simulink library "INT_TIntkVUs_DD"  (R2016b)
settings: Solver=VariableStepAuto  StartTime=0.0  StopTime=10.0  RelTol=1e-3
settings Model: Creator=Administrator  LastModifiedBy=Administrator

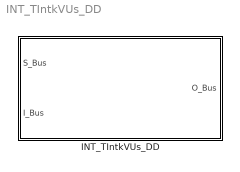
== system INT_TIntkVUs_DD ==
  INT_TIntkVUs_DD : Subsystem

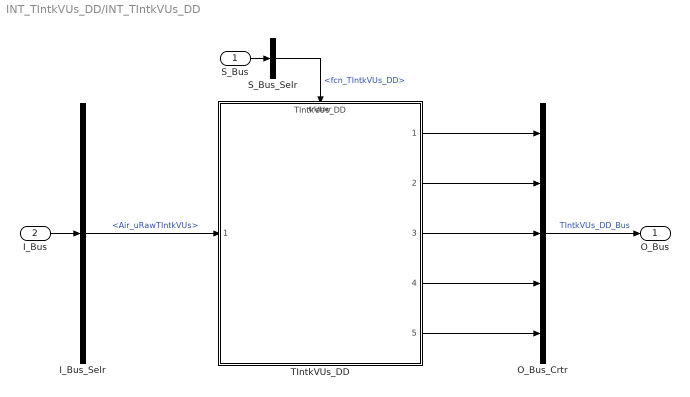
== system INT_TIntkVUs_DD/INT_TIntkVUs_DD ==
  S_Bus : Inport
  I_Bus : Inport  Port=2
  I_Bus_Selr : BusSelector  OutputSignals=Air_uRawTIntkVUs
  O_Bus_Crtr : BusCreator  Inputs=5
  S_Bus_Selr : BusSelector  OutputSignals=fcn_TIntkVUs_DD
  TIntkVUs_DD : ModelReference  ModelNameDialog=TIntkVUs_DD  SimulationMode=Normal  ModelReferenceVersion=1.12  TriggerPortName=function  TriggerPortTriggerType=function-call  TriggerPortStatesWhenEnabling=held
  O_Bus : Outport
  wires:
  S_Bus_Selr/1 -> TIntkVUs_DD/Trigger  "<fcn_TIntkVUs_DD>"
  S_Bus/1 -> S_Bus_Selr/1
  I_Bus/1 -> I_Bus_Selr/1
  I_Bus_Selr/1 -> TIntkVUs_DD/1  "<Air_uRawTIntkVUs>"
  O_Bus_Crtr/1 -> O_Bus/1  "TIntkVUs_DD_Bus"
  TIntkVUs_DD/1 -> O_Bus_Crtr/1
  TIntkVUs_DD/2 -> O_Bus_Crtr/2
  TIntkVUs_DD/3 -> O_Bus_Crtr/3
  TIntkVUs_DD/4 -> O_Bus_Crtr/4
  TIntkVUs_DD/5 -> O_Bus_Crtr/5
